simulink model "PID"  (R2020b)
settings: Solver=VariableStepAuto  StartTime=0.0  StopTime=st  RelTol=1e-3
values from neighbouring files (symbols this model uses):
  DEN_P = str2num(get(handles.den_p_text,'string'))    [PID_diff.m]
  dis_in_amp = str2num(get(handles.dis_in_amp_text,'string'))    [PID_diff.m]
  dis_out_amp = str2num(get(handles.dis_out_amp_text,'string'))    [PID_diff.m]
  kd = str2num(get(handles.kd_text,'string'))    [PID_diff.m]
  ki = str2num(get(handles.ki_text,'string'))    [PID_diff.m]
  kp = str2num(get(handles.kp_text,'string'))    [PID_diff.m]    (also in auto_cont_final_proj.m = dcgain(g))
  noise_amp = str2num(get(handles.noise_amp_text,'string'))    [PID_diff.m]
  noise_freq = str2num(get(handles.noise_freq_text,'string'))    [PID_diff.m]
  noise_var = str2num(get(handles.noise_var_text,'string'))    [PID_diff.m]
  NUM_P = str2num(get(handles.num_p_text,'string'))    [PID_diff.m]
undefined symbols (not defined in the file or in its folder): dis_in_time, dis_out_time, sp
libraries: pid_lib x1
settings Model: Creator=AbdelRaHmaN ShRieF  LastModifiedBy=AbdelRaHmaN ShRieF
settings DataIOCC: SignalLogging=off  DSMLogging=off  ReturnWorkspaceOutputs=off
settings DebuggingCC: SFMachineParentedDataDiag=error

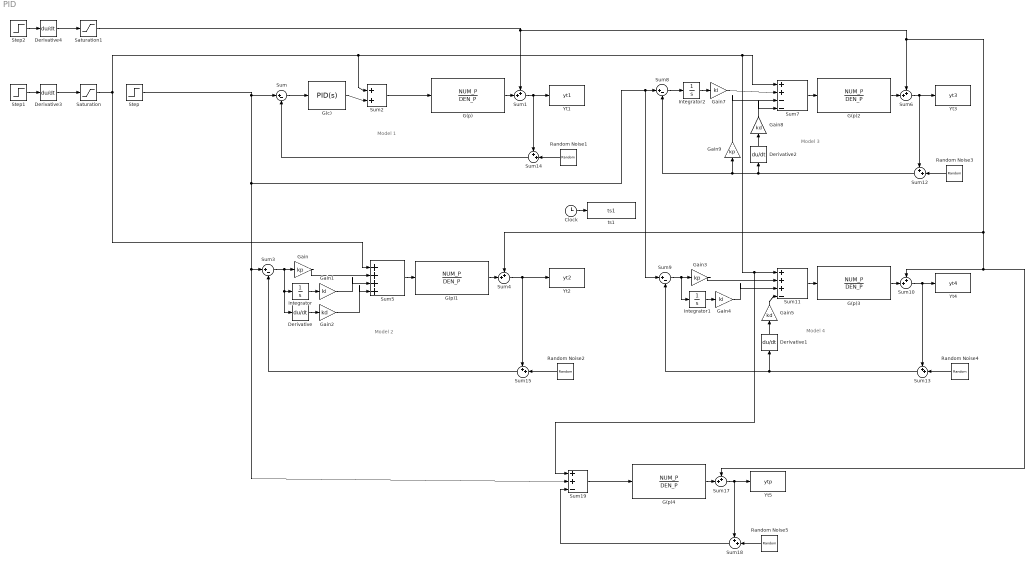
== system PID ==
  note: Model 1
  note: Model 3
  note: Model 4
  note: Model 2
  Clock : Clock
      settings: Tag=Clock  AttributesFormatString=%<Tag>
  Derivative{,1..4} (5 alike) : Derivative
  G(c) : pid_lib/PID Controller  Controller=PID  Form=Parallel  TimeDomain=Continuous-time  UseExternalTs=off  SampleTime=-1  IntegratorMethod=Forward Euler  ControllerParametersSource=internal  P=kp  I=ki  D=kd  UseFilter=on  N=100  TunerSelectOption=Transfer Function Based (PID Tuner App)  InitialConditionSource=internal  InitialConditionForIntegrator=0  InitialConditionForFilter=0  DifferentiatorICPrevScaledInput=0  ExternalReset=none  TrackingMode=off  Kt=1  LimitOutput=off  SatLimitsSource=internal  UpperSaturationLimit=inf  LowerSaturationLimit=-inf  LinearizeAsGain=on  AntiWindupMode=none  Kb=1  POutMin=[]  POutMax=[]  IOutMin=[]  IOutMax=[]  DOutMin=[]  DOutMax=[]  NOutMin=[]  NOutMax=[]  SumOutMin=[]  SumOutMax=[]  SaturationOutMin=[]  SaturationOutMax=[]  PParamMin=[]  PParamMax=[]  IParamMin=[]  IParamMax=[]  DParamMin=[]  DParamMax=[]  NParamMin=[]  NParamMax=[]  KbParamMin=[]  KbParamMax=[]  KtParamMin=[]  KtParamMax=[]  KbOutMin=[]  KbOutMax=[]  KtOutMin=[]  KtOutMax=[]  IntegratorOutMin=[]  IntegratorOutMax=[]  FilterOutMin=[]  FilterOutMax=[]  SumI1OutMin=[]  SumI1OutMax=[]  SumI2OutMin=[]  SumI2OutMax=[]  SumI3OutMin=[]  SumI3OutMax=[]  SumI4OutMin=[]  SumI4OutMax=[]  SumDOutMin=[]  SumDOutMax=[]  DifferentiatorOutMin=[]  DifferentiatorOutMax=[]  FilterDiffOutCoefMin=[]  FilterDiffOutCoefMax=[]  ReciprocalOutMin=[]  ReciprocalOutMax=[]  SumDenOutMin=[]  SumDenOutMax=[]  SumNumOutMin=[]  SumNumOutMax=[]  DivideOutMin=[]  DivideOutMax=[]  UdiffTsProdOutMin=[]  UdiffTsProdOutMax=[]  NTsProdOutMin=[]  NTsProdOutMax=[]  UintegralTsProdOutMin=[]  UintegralTsProdOutMax=[]  UngainTsProdOutMin=[]  UngainTsProdOutMax=[]  IntegratorContinuousStateAttributes=''  IntegratorStateMustResolveToSignalObject=off  IntegratorRTWStateStorageClass=Auto  FilterContinuousStateAttributes=''  FilterStateMustResolveToSignalObject=off  FilterRTWStateStorageClass=Auto  ParallelPVariant=InternalParameters  IdealPVariant=Disabled  IVariant=InternalParameters  DVariant=InternalParameters  IntegratorVariant=Continuous  SatVariant=Disabled  AWVariant=Passthrough  PCopyVariant=Disabled  TRVariant=Disabled  FdbkBlocksVariant=Forward  IdealPFdbkVariant=Disabled  SatFdbkVariant=Disabled  DerivativeFilterVariant=ContFilter  NVariant=InternalParameters  NCopyVariant=Disabled  FilterICVariant=InternalICsFilter  IntegratorICVariant=InternalICs  ExternalResetVariant=Disabled  TRSumVariant=Passthrough  SumFdbkVariant=Disabled  SumVariant=Sum_PID  TsampFilterVariant=InternalTs  TsampNgainVariant=Passthrough  TsampIntegralVariant=Passthrough  ExternalSaturationOutDataTypeStr=Inherit: Same as second input
  G(p){,1..4} (5 alike) : TransferFcn  Numerator=NUM_P  Denominator=DEN_P
  Gain : Gain  Gain=kp
  Gain1 : Gain  Gain=ki
  Gain2 : Gain  Gain=kd
  Gain3 : Gain  Gain=kp
  Gain4 : Gain  Gain=ki
  Gain5 : Gain  Gain=kd
  Gain7 : Gain  Gain=ki
  Gain8 : Gain  Gain=kd
  Gain9 : Gain  Gain=kp
  Integrator : Integrator
  Integrator1 : Integrator
  Integrator2 : Integrator
  Random Noise{1..5} (5 alike) : RandomNumber  Mean=noise_amp  Variance=noise_var  SampleTime=1/noise_freq
  Saturation : Saturate  UpperLimit=dis_in_amp  LowerLimit=0
  Saturation1 : Saturate  UpperLimit=dis_out_amp  LowerLimit=0
  Step : Step  After=sp  SampleTime=0
      settings: AttributesFormatString=%<Name>
  Step1 : Step  Time=dis_in_time  SampleTime=0
      settings: AttributesFormatString=%<Name>
  Step2 : Step  Time=dis_out_time  SampleTime=0
      settings: AttributesFormatString=%<Name>
  Sum{,3,8..9} (4 alike) : Sum  Inputs=|+-
  Sum{1..2,4,6,10,12..15,17..18} (11 alike) : Sum  Inputs=++|
  Sum11 : Sum  Inputs=+++-|
  Sum19 : Sum  Inputs=++-|
  Sum5 : Sum  Inputs=++++|
  Sum7 : Sum  Inputs=++--|
  Yt1 : ToWorkspace  VariableName=yt1  SampleTime=-1
      settings: Save2DSignal=2-D array (concatenate along first dimension)
  Yt2 : ToWorkspace  VariableName=yt2  SampleTime=-1
      settings: Save2DSignal=2-D array (concatenate along first dimension)
  Yt3 : ToWorkspace  VariableName=yt3  SampleTime=-1
      settings: Save2DSignal=2-D array (concatenate along first dimension)
  Yt4 : ToWorkspace  VariableName=yt4  SampleTime=-1
      settings: Save2DSignal=2-D array (concatenate along first dimension)
  Yt5 : ToWorkspace  VariableName=ytp  SampleTime=-1
      settings: Save2DSignal=2-D array (concatenate along first dimension)
  ts1 : ToWorkspace  VariableName=ts1  SampleTime=-1
      settings: Save2DSignal=2-D array (concatenate along first dimension)
  wires:
  Sum/1 -> G(c)/1
  G(c)/1 -> Sum2/2
  Sum2/1 -> G(p)/1
  G(p)/1 -> Sum1/2
  Clock/1 -> ts1/1
  Saturation/1 -> Sum19/1, Sum11/1, Sum7/1, Sum2/1, Sum5/1
  Sum4/1 -> Sum15/1, Yt2/1
  G(p)1/1 -> Sum4/2
  Saturation1/1 -> Sum1/1, Sum4/1, Sum10/1, Sum17/1, Sum6/1
  Sum3/1 -> Derivative/1, Integrator/1, Gain/1
  Integrator/1 -> Gain1/1
  Derivative/1 -> Gain2/1
  Sum5/1 -> G(p)1/1
  Gain1/1 -> Sum5/3
  Gain/1 -> Sum5/2
  Gain2/1 -> Sum5/4
  Sum11/1 -> G(p)3/1
  Derivative1/1 -> Gain5/1
  Sum9/1 -> Integrator1/1, Gain3/1
  Sum10/1 -> Yt4/1, Sum13/1
  G(p)3/1 -> Sum10/2
  Gain4/1 -> Sum11/3
  Gain3/1 -> Sum11/2
  Gain5/1 -> Sum11/4
  Integrator1/1 -> Gain4/1
  Integrator2/1 -> Gain7/1
  Sum6/1 -> Sum12/1, Yt3/1
  G(p)2/1 -> Sum6/2
  Sum8/1 -> Integrator2/1
  Derivative2/1 -> Gain8/1
  Gain8/1 -> Sum7/4
  Sum7/1 -> G(p)2/1
  Gain9/1 -> Sum7/3
  Gain7/1 -> Sum7/2
  Random Noise3/1 -> Sum12/2
  Sum12/1 -> Derivative2/1, Gain9/1, Sum8/2
  Random Noise4/1 -> Sum13/2
  Sum13/1 -> Sum9/2, Derivative1/1
  Sum1/1 -> Sum14/1, Yt1/1
  Random Noise1/1 -> Sum14/2
  Sum14/1 -> Sum/2
  Random Noise2/1 -> Sum15/2
  Sum15/1 -> Sum3/2
  Random Noise5/1 -> Sum18/2
  Step/1 -> Sum19/2, Sum3/1, Sum9/1, Sum8/1, Sum/1
  G(p)4/1 -> Sum17/2
  Sum17/1 -> Sum18/1, Yt5/1
  Sum19/1 -> G(p)4/1
  Sum18/1 -> Sum19/3
  Step1/1 -> Derivative3/1
  Step2/1 -> Derivative4/1
  Derivative3/1 -> Saturation/1
  Derivative4/1 -> Saturation1/1
